simulink model "unstable"  (R2018b)
settings: Solver=VariableStepAuto  StartTime=0.0  StopTime=50  RelTol=1e-3
libraries: cstblocks x2
settings Model: Creator=Oguz  LastModifiedBy=Oguz

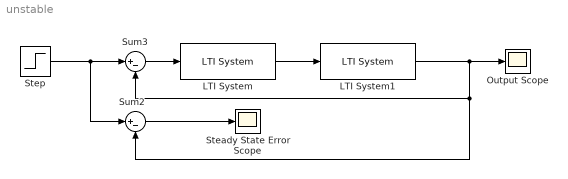
== system unstable ==
  LTI System : cstblocks/LTI System  sys=C  IC=[]
  LTI System1 : cstblocks/LTI System  sys=P  IC=[]
  "Output Scope " : Scope
      settings: Description=Output Scope
  Steady State Error Scope : Scope
  Step : Step  SampleTime=0
  Sum2 : Sum  Inputs=|+-
  Sum3 : Sum  Inputs=|+-
  wires:
  LTI System1/1 -> "Output Scope "/1, Sum2/2, Sum3/2
  Sum2/1 -> Steady State Error Scope/1
  Step/1 -> Sum2/1, Sum3/1
  LTI System/1 -> LTI System1/1
  Sum3/1 -> LTI System/1
